simulink model "sampleModel2438"  (R2017a)
settings: Solver=VariableStepAuto  StartTime=0.0  StopTime=10.0  RelTol=1e-3
undefined symbols (not defined in the file or in its folder): DiscIntNeverNeededParam, sigbuilder_block
libraries: simulink x299
(part 1 of 5)
settings Model: Creator=cyfuzz  LastModifiedBy=cyfuzz

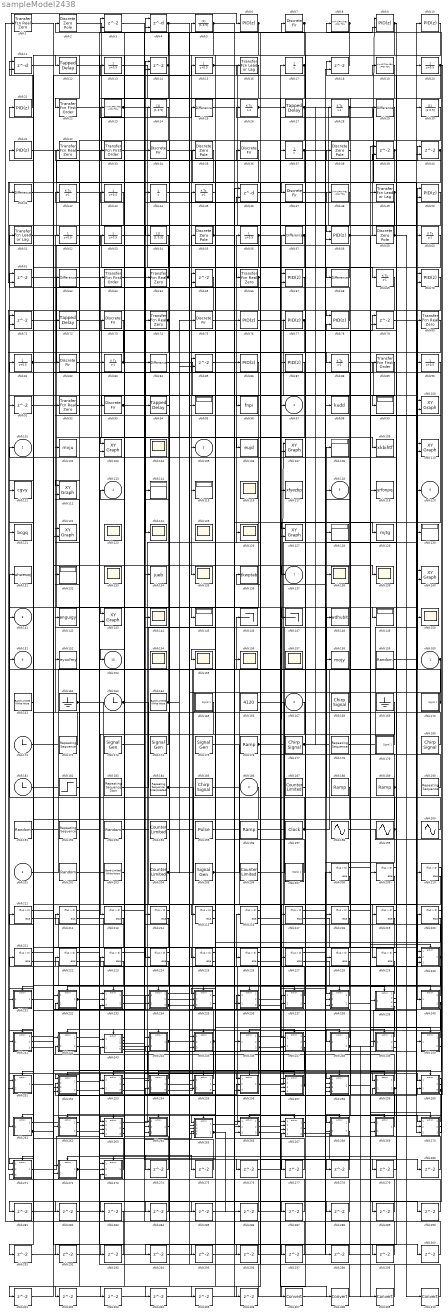
== system sampleModel2438 ==
  cfblk160 : Inport
  cfblk167 : Inport  Port=2
  cfblk186 : Inport  Port=3
  cfblk201 : Inport  Port=4
  cfblk{1,32,64,66,74,80,92} (7 alike) : simulink/Discrete/Transfer Fcn Real Zero  ZeroZ=0.75  ICPrevInput=0.0  DoSatur=off
      settings: SourceProductName=Simulink  SourceProductBaseCode=SL
  cfblk{6,10,21,31,76..77,86..87} (8 alike) : simulink/Continuous/PID Controller  Controller=PID  TimeDomain=Discrete-time  SampleTime=1  IntegratorMethod=Forward Euler  FilterMethod=Forward Euler  Form=Parallel  UseFilter=on  ControllerParametersSource=internal  P=1  I=1  D=0  N=100  InitialConditionSource=internal  InitialConditionForIntegrator=0  InitialConditionForFilter=0  ExternalReset=none  LimitOutput=off  UpperSaturationLimit=inf  LowerSaturationLimit=-inf  LinearizeAsGain=off  AntiWindupMode=none  Kb=1  TrackingMode=off  Kt=1  PParamMin=[]  PParamMax=[]  IParamMin=[]  IParamMax=[]  DParamMin=[]  DParamMax=[]  NParamMin=[]  NParamMax=[]  KbParamMin=[]  KbParamMax=[]  KtParamMin=[]  KtParamMax=[]  POutMin=[]  POutMax=[]  IOutMin=[]  IOutMax=[]  DOutMin=[]  DOutMax=[]  NOutMin=[]  NOutMax=[]  KbOutMin=[]  KbOutMax=[]  KtOutMin=[]  KtOutMax=[]  IntegratorOutMin=[]  IntegratorOutMax=[]  FilterOutMin=[]  FilterOutMax=[]  SumOutMin=[]  SumOutMax=[]  SumI1OutMin=[]  SumI1OutMax=[]  SumI2OutMin=[]  SumI2OutMax=[]  SumI3OutMin=[]  SumI3OutMax=[]  SumDOutMin=[]  SumDOutMax=[]  SaturationOutMin=[]  SaturationOutMax=[]  IntegratorContinuousStateAttributes=''  IntegratorStateMustResolveToSignalObject=off  IntegratorRTWStateStorageClass=Auto  FilterContinuousStateAttributes=''  FilterStateMustResolveToSignalObject=off  FilterRTWStateStorageClass=Auto  DifferentiatorICPrevScaledInput=0  DifferentiatorOutMin=[]  DifferentiatorOutMax=[]  InitialConditionSetting=State (most efficient)
  cfblk{100,103,107,110,112,122,127,140,143} (9 alike) : simulink/Sinks/XY Graph  xmin=-1  xmax=1  ymin=-1  ymax=1  st=-1
  cfblk102 : ToFile  Filename=mvju  SaveFormat=Timeseries
  cfblk{104,116,123..126,133,135,138..139,144,150,154..157} (16 alike) : Scope
      cfblk104 settings: Floating=on
      cfblk116 settings: Floating=on
      cfblk123 settings: Floating=on
      cfblk125 settings: Floating=on
      cfblk133 settings: Floating=on
      cfblk154 settings: Floating=on
      cfblk157 settings: Floating=on
  cfblk106 : ToFile  Filename=eujd  SaveFormat=Timeseries
  cfblk{95,99,108,114..115,128,130,132,145,149} (10 alike) : Display
  cfblk109 : ToWorkspace  VariableName=xkbihtf  SaveFormat=Timeseries  SampleTime=-1
  cfblk11 : Delay  DelayLengthSource=Input port  SampleTime=1
      settings: InputPortMap=u0,p1
  cfblk111 : ToFile  Filename=cgvy  SaveFormat=Timeseries
  cfblk117 : ToWorkspace  VariableName=xfyezbp  SaveFormat=Timeseries  SampleTime=-1
  cfblk119 : ToWorkspace  VariableName=yrfonpq  SaveFormat=Timeseries  SampleTime=-1
  cfblk{12,27,72,94} (4 alike) : simulink/Discrete/Tapped Delay  vinit=0.0  samptime=-1  NumDelays=1  DelayOrder=Oldest  includeCurrent=off
  cfblk121 : ToFile  Filename=bcgq  SaveFormat=Timeseries
  cfblk129 : ToFile  Filename=mjtg  SaveFormat=Timeseries
  cfblk{13,15,20,43,52..53,56,81,90} (9 alike) : DiscreteTransferFcn  SampleTime=1
  cfblk131 : ToWorkspace  VariableName=whweswj  SaveFormat=Timeseries  SampleTime=-1
  cfblk134 : ToFile  Filename=jueb  SaveFormat=Timeseries
  cfblk136 : ToWorkspace  VariableName=tkwpteb  SaveFormat=Timeseries  SampleTime=-1
  cfblk{3,14,18,39..40,61,65,71,79,85} (10 alike) : Delay  ShowEnablePort=on  SampleTime=1
      settings: InputPortMap=u0,e6
  cfblk142 : ToWorkspace  VariableName=enguigy  SaveFormat=Timeseries  SampleTime=-1
  cfblk146 : Terminator
  cfblk147 : Terminator
  cfblk148 : ToWorkspace  VariableName=wdhubit  SaveFormat=Timeseries  SampleTime=-1
  cfblk152 : ToWorkspace  VariableName=eyoxfmy  SaveFormat=Timeseries  SampleTime=-1
  cfblk158 : ToFile  Filename=mojy  SaveFormat=Timeseries
  cfblk{159,191,193,202} (4 alike) : UniformRandomNumber  SampleTime=0.1
  cfblk16 : simulink/Discrete/Transfer Fcn Lead or Lag  PoleZ=0.95  ZeroZ=0.75  ICPrevOutput=0.0  ICPrevInput=0.0  DoSatur=off
      settings: SourceProductName=Simulink  SourceProductBaseCode=SL
  cfblk161 : simulink/Sources/Band-Limited White Noise  Cov=[0.1]  Ts=0.1  seed=[23341]
  cfblk162 : Ground
  cfblk163 : Clock
  cfblk164 : simulink/Sources/Band-Limited White Noise  Cov=[0.1]  Ts=0.1  seed=[23341]
  cfblk165 : Subsystem  Tag=STV Subsys  LoadFcn=sigbuilder_block('load');  StartFcn=sigbuilder_block('start');  StopFcn=sigbuilder_block('stop');  ClipboardFcn=sigbuilder_block('clipboard');  mask(Sigbuilder block){tuvar=[0:10]}
      mask help: Simulink:masks:SigbuilderBlock_MD
      mask init:
      | if ~strcmp(get_param(bdroot(gcbh),'SimulationStatus'),'stopped') tuvar = sigbuilder_block('maskInit'); end
      settings: CopyFcn=sigbuilder_block('copy');  DeleteFcn=sigbuilder_block('delete');  ModelCloseFcn=sigbuilder_block('modelClose');  PreSaveFcn=sigbuilder_block('preSave');  PauseFcn=sigbuilder_block('pause');  ContinueFcn=sigbuilder_block('continue');  NameChangeFcn=sigbuilder_block('namechange');  OpenFcn=sigbuilder_block('open',[437.6 199.2 550.4 400 ]);  CloseFcn=sigbuilder_block('close');
      mask Display: plot(0, 0, 100, 100,[2, 2, 32, 32, 2], [68, 8, 8, 68, 68],[32, 2], [38, 38], [32, 19, 2],[53, 60, 44], [32, 17, 17, 2],[16, 16, 31, 31]);txt = getActiveGroup(gcbh);text(2, 100, txt,'verticalAlignment', 'top');
  cfblk166 : Constant  Value=4120
  cfblk{168,177,180,185} (4 alike) : simulink/Sources/Chirp Signal  f1=0.1  T=100  f2=1
  cfblk169 : Ground
  cfblk17 : UnitDelay
  cfblk170 : Subsystem  Tag=STV Subsys  LoadFcn=sigbuilder_block('load');  StartFcn=sigbuilder_block('start');  StopFcn=sigbuilder_block('stop');  ClipboardFcn=sigbuilder_block('clipboard');  mask(Sigbuilder block){tuvar=[0:10]}
      mask help: Simulink:masks:SigbuilderBlock_MD
      mask init:
      | if ~strcmp(get_param(bdroot(gcbh),'SimulationStatus'),'stopped') tuvar = sigbuilder_block('maskInit'); end
      settings: CopyFcn=sigbuilder_block('copy');  DeleteFcn=sigbuilder_block('delete');  ModelCloseFcn=sigbuilder_block('modelClose');  PreSaveFcn=sigbuilder_block('preSave');  PauseFcn=sigbuilder_block('pause');  ContinueFcn=sigbuilder_block('continue');  NameChangeFcn=sigbuilder_block('namechange');  OpenFcn=sigbuilder_block('open',[437.6 199.2 550.4 400 ]);  CloseFcn=sigbuilder_block('close');
      mask Display: plot(0, 0, 100, 100,[2, 2, 32, 32, 2], [68, 8, 8, 68, 68],[32, 2], [38, 38], [32, 19, 2],[53, 60, 44], [32, 17, 17, 2],[16, 16, 31, 31]);txt = getActiveGroup(gcbh);text(2, 100, txt,'verticalAlignment', 'top');
  cfblk171 : Clock
  cfblk{172,178,190,192} (4 alike) : simulink/Sources/Repeating Sequence  rep_seq_t=[0 2]  rep_seq_y=[0 2]
  cfblk{173..175,205} (4 alike) : SignalGenerator  Units=rad/sec
  cfblk{176,188..189,196} (4 alike) : simulink/Sources/Ramp  slope=1  start=0  X0=0
  cfblk179 : Subsystem  Tag=STV Subsys  LoadFcn=sigbuilder_block('load');  StartFcn=sigbuilder_block('start');  StopFcn=sigbuilder_block('stop');  ClipboardFcn=sigbuilder_block('clipboard');  mask(Sigbuilder block){tuvar=[0:10]}
      mask help: Simulink:masks:SigbuilderBlock_MD
      mask init:
      | if ~strcmp(get_param(bdroot(gcbh),'SimulationStatus'),'stopped') tuvar = sigbuilder_block('maskInit'); end
      settings: CopyFcn=sigbuilder_block('copy');  DeleteFcn=sigbuilder_block('delete');  ModelCloseFcn=sigbuilder_block('modelClose');  PreSaveFcn=sigbuilder_block('preSave');  PauseFcn=sigbuilder_block('pause');  ContinueFcn=sigbuilder_block('continue');  NameChangeFcn=sigbuilder_block('namechange');  OpenFcn=sigbuilder_block('open',[437.6 199.2 550.4 400 ]);  CloseFcn=sigbuilder_block('close');
      mask Display: plot(0, 0, 100, 100,[2, 2, 32, 32, 2], [68, 8, 8, 68, 68],[32, 2], [38, 38], [32, 19, 2],[53, 60, 44], [32, 17, 17, 2],[16, 16, 31, 31]);txt = getActiveGroup(gcbh);text(2, 100, txt,'verticalAlignment', 'top');
  cfblk181 : Clock
  cfblk182 : Step  After=81  SampleTime=0
  cfblk183 : simulink/Sources/Repeating Sequence Stair  OutValues=[3 1 4 2 1].'  tsamp=-1  OutMin=[]  OutMax=[]  OutDataTypeStr=double  OutputDataTypeScalingMode=double  OutDataType=fixdt(0,8)  ConRadixGroup=Best Precision: Vector-wise  OutScaling=2^-12
  cfblk184 : simulink/Sources/Repeating Sequence Interpolated  OutValues=[3 1 4 2 1].'  TimeValues=[0 0.1 0.5 0.6 1].'  LookUpMeth=Interpolation-Use End Values  tsamp=0.01  OutMin=[]  OutMax=[]  OutDataTypeStr=double  OutputDataTypeScalingMode=double  OutDataType=fixdt(0,8)  OutScaling=2^-10
  cfblk{187,194,204,206} (4 alike) : simulink/Sources/Counter Limited  uplimit=7  tsamp=-1
  cfblk{8,19,23,48} (4 alike) : DiscreteStateSpace
  cfblk195 : DiscretePulseGenerator  PulseType=Time based  Period=10  PulseWidth=5
  cfblk197 : DigitalClock
  cfblk198 : Sin  SampleTime=0
  cfblk199 : Sin  SampleTime=0
  cfblk{2,35,38,55,59} (5 alike) : DiscreteZeroPole  Poles=[0 0.5]  Gain=1
  cfblk200 : Sin  SampleTime=0
  cfblk203 : simulink/Sources/Band-Limited White Noise  Cov=[0.1]  Ts=0.1  seed=[23341]
  cfblk207 : Subsystem  Tag=STV Subsys  LoadFcn=sigbuilder_block('load');  StartFcn=sigbuilder_block('start');  StopFcn=sigbuilder_block('stop');  ClipboardFcn=sigbuilder_block('clipboard');  mask(Sigbuilder block){tuvar=[0:10]}
      mask help: Simulink:masks:SigbuilderBlock_MD
      mask init:
      | if ~strcmp(get_param(bdroot(gcbh),'SimulationStatus'),'stopped') tuvar = sigbuilder_block('maskInit'); end
      settings: CopyFcn=sigbuilder_block('copy');  DeleteFcn=sigbuilder_block('delete');  ModelCloseFcn=sigbuilder_block('modelClose');  PreSaveFcn=sigbuilder_block('preSave');  PauseFcn=sigbuilder_block('pause');  ContinueFcn=sigbuilder_block('continue');  NameChangeFcn=sigbuilder_block('namechange');  OpenFcn=sigbuilder_block('open',[437.6 199.2 550.4 400 ]);  CloseFcn=sigbuilder_block('close');
      mask Display: plot(0, 0, 100, 100,[2, 2, 32, 32, 2], [68, 8, 8, 68, 68],[32, 2], [38, 38], [32, 19, 2],[53, 60, 44], [32, 17, 17, 2],[16, 16, 31, 31]);txt = getActiveGroup(gcbh);text(2, 100, txt,'verticalAlignment', 'top');
  cfblk{208..229} (22 alike) : If  SampleTime=1
  cfblk{22,33,63,89} (4 alike) : simulink/Discrete/Transfer Fcn First Order  PoleZ=0.95  ICPrevOutput=0.0  DoSatur=off
      settings: SourceProductName=Simulink
  cfblk230 : Subsystem  TreatAsAtomicUnit=on
  cfblk231 : Subsystem  TreatAsAtomicUnit=on
  cfblk232 : Subsystem  TreatAsAtomicUnit=on
  cfblk233 : Subsystem  TreatAsAtomicUnit=on
  cfblk234 : Subsystem  TreatAsAtomicUnit=on
  cfblk235 : Subsystem  TreatAsAtomicUnit=on
  cfblk236 : Subsystem  TreatAsAtomicUnit=on
  cfblk237 : Subsystem  TreatAsAtomicUnit=on
  cfblk238 : Subsystem  TreatAsAtomicUnit=on
  cfblk239 : Subsystem  TreatAsAtomicUnit=on
  cfblk{5,24,30,54} (4 alike) : DiscreteFilter  SampleTime=1
  cfblk240 : Subsystem  TreatAsAtomicUnit=on
  cfblk241 : Subsystem  TreatAsAtomicUnit=on
  cfblk242 : Subsystem  TreatAsAtomicUnit=on
  cfblk243 : Subsystem  TreatAsAtomicUnit=on
  cfblk244 : Subsystem  TreatAsAtomicUnit=on
  cfblk245 : Subsystem  TreatAsAtomicUnit=on
  cfblk246 : Subsystem  TreatAsAtomicUnit=on
  cfblk247 : Subsystem  TreatAsAtomicUnit=on
  cfblk248 : Subsystem  TreatAsAtomicUnit=on
  cfblk249 : Subsystem  TreatAsAtomicUnit=on
  cfblk{25,29,41,57,62,68,84} (7 alike) : simulink/Discrete/Difference  ICPrevInput=0.0  OutMin=[]  OutMax=[]  OutDataTypeStr=Inherit: Inherit via back propagation  OutDataType=fixdt(1, 16)  OutScaling=2^-10  DoSatur=off
  cfblk250 : Subsystem  TreatAsAtomicUnit=on
  cfblk251 : Subsystem  TreatAsAtomicUnit=on
  cfblk252 : Subsystem  TreatAsAtomicUnit=on
  cfblk253 : Subsystem  TreatAsAtomicUnit=on
  cfblk254 : Subsystem  TreatAsAtomicUnit=on
  cfblk255 : Subsystem  TreatAsAtomicUnit=on
  cfblk256 : Subsystem  TreatAsAtomicUnit=on
  cfblk257 : Subsystem  TreatAsAtomicUnit=on
  cfblk258 : Subsystem  TreatAsAtomicUnit=on
  cfblk259 : Subsystem  TreatAsAtomicUnit=on
  cfblk{26,28,42,45,60,69,83,88} (8 alike) : DiscreteIntegrator  InitialConditionSetting=State (most efficient)  ICPrevOutput=DiscIntNeverNeededParam  ICPrevScaledInput=DiscIntNeverNeededParam
  cfblk260 : Subsystem  TreatAsAtomicUnit=on
  cfblk261 : Subsystem  TreatAsAtomicUnit=on
  cfblk262 : Subsystem  TreatAsAtomicUnit=on
  cfblk263 : Subsystem  TreatAsAtomicUnit=on
  cfblk264 : Subsystem  TreatAsAtomicUnit=on
  cfblk265 : Subsystem  TreatAsAtomicUnit=on
  cfblk266 : Subsystem  TreatAsAtomicUnit=on
  cfblk267 : Subsystem  TreatAsAtomicUnit=on
  cfblk268 : Subsystem  TreatAsAtomicUnit=on
  cfblk269 : Subsystem  TreatAsAtomicUnit=on
  cfblk270 : Subsystem  TreatAsAtomicUnit=on
  cfblk271 : Subsystem  TreatAsAtomicUnit=on
  cfblk272 : Subsystem  TreatAsAtomicUnit=on
  cfblk273 : Subsystem  TreatAsAtomicUnit=on
  cfblk{91,274..306} (34 alike) : Delay  SampleTime=1
  cfblk{307..310} (4 alike) : DataTypeConversion
  cfblk{7,34,36,47,73,75,82,93} (8 alike) : DiscreteFir  SampleTime=1
  cfblk37 : UnitDelay
  cfblk4 : Delay  DelayLengthSource=Input port  SampleTime=1
      settings: InputPortMap=u0,p1
  cfblk44 : UnitDelay
  cfblk46 : Delay  DelayLengthSource=Input port  SampleTime=1
      settings: InputPortMap=u0,p1
  cfblk49 : simulink/Discrete/Transfer Fcn Lead or Lag  PoleZ=0.95  ZeroZ=0.75  ICPrevOutput=0.0  ICPrevInput=0.0  DoSatur=off
      settings: SourceProductName=Simulink  SourceProductBaseCode=SL
  cfblk{9,50,58,67,70,78} (6 alike) : simulink/Continuous/PID Controller (2DOF)  Controller=PID  TimeDomain=Discrete-time  SampleTime=1  IntegratorMethod=Forward Euler  FilterMethod=Forward Euler  Form=Parallel  UseFilter=on  ControllerParametersSource=internal  P=1  I=1  D=0  N=100  b=1  c=1  InitialConditionSource=internal  InitialConditionForIntegrator=0  InitialConditionForFilter=0  ExternalReset=none  LimitOutput=off  UpperSaturationLimit=inf  LowerSaturationLimit=-inf  LinearizeAsGain=off  AntiWindupMode=none  Kb=1  TrackingMode=off  Kt=1  PParamMin=[]  PParamMax=[]  IParamMin=[]  IParamMax=[]  DParamMin=[]  DParamMax=[]  NParamMin=[]  NParamMax=[]  bParamMin=[]  bParamMax=[]  cParamMin=[]  cParamMax=[]  KbParamMin=[]  KbParamMax=[]  KtParamMin=[]  KtParamMax=[]  POutMin=[]  POutMax=[]  IOutMin=[]  IOutMax=[]  DOutMin=[]  DOutMax=[]  NOutMin=[]  NOutMax=[]  bOutMin=[]  bOutMax=[]  cOutMin=[]  cOutMax=[]  KbOutMin=[]  KbOutMax=[]  KtOutMin=[]  KtOutMax=[]  IntegratorOutMin=[]  IntegratorOutMax=[]  FilterOutMin=[]  FilterOutMax=[]  SumOutMin=[]  SumOutMax=[]  Sum1OutMin=[]  Sum1OutMax=[]  Sum2OutMin=[]  Sum2OutMax=[]  Sum3OutMin=[]  Sum3OutMax=[]  SumI1OutMin=[]  SumI1OutMax=[]  SumI2OutMin=[]  SumI2OutMax=[]  SumI3OutMin=[]  SumI3OutMax=[]  SumDOutMin=[]  SumDOutMax=[]  SaturationOutMin=[]  SaturationOutMax=[]  IntegratorContinuousStateAttributes=''  IntegratorStateMustResolveToSignalObject=off  IntegratorRTWStateStorageClass=Auto  FilterContinuousStateAttributes=''  FilterStateMustResolveToSignalObject=off  FilterRTWStateStorageClass=Auto  DifferentiatorICPrevScaledInput=0  DifferentiatorOutMin=[]  DifferentiatorOutMax=[]  InitialConditionSetting=State (most efficient)
  cfblk51 : simulink/Discrete/Transfer Fcn Lead or Lag  PoleZ=0.95  ZeroZ=0.75  ICPrevOutput=0.0  ICPrevInput=0.0  DoSatur=off
      settings: SourceProductName=Simulink  SourceProductBaseCode=SL
  cfblk96 : ToFile  Filename=fnpi  SaveFormat=Timeseries
  cfblk98 : ToFile  Filename=kudd  SaveFormat=Timeseries
  cfblk97 : Outport
  cfblk101 : Outport  Port=2
  cfblk105 : Outport  Port=3
  cfblk113 : Outport  Port=4
  cfblk118 : Outport  Port=5
  cfblk120 : Outport  Port=6
  cfblk137 : Outport  Port=7
  cfblk141 : Outport  Port=8
  cfblk151 : Outport  Port=9
  cfblk153 : Outport  Port=10
  wires:
  cfblk43/1 -> cfblk261/1(cfblk1)
  cfblk10/1 -> cfblk135/1
  cfblk246/1(cfblk2) -> cfblk259/1(cfblk1)
  cfblk200/1 -> cfblk108/1
  cfblk83/1 -> cfblk63/1, cfblk258/4(cfblk15)
  cfblk18/1 -> cfblk12/1
  cfblk238/1(cfblk2) -> cfblk14/1
  cfblk237/1(cfblk2) -> cfblk55/1
  cfblk198/1 -> cfblk50/1
  cfblk273/1(cfblk2) -> cfblk71/1
  cfblk58/1 -> cfblk9/1, cfblk230/3(cfblk14), cfblk290/1
  cfblk239/1(cfblk2) -> cfblk57/1
  cfblk45/1 -> cfblk145/1
  cfblk51/1 -> cfblk40/1
  cfblk16/1 -> cfblk155/1
  cfblk4/1 -> cfblk88/1, cfblk293/1
  cfblk194/1 -> cfblk50/2
  cfblk52/1 -> cfblk124/1
  cfblk23/1 -> cfblk69/1, cfblk258/1(cfblk1)
  cfblk239/2(cfblk14) -> cfblk71/2
  cfblk166/1 -> cfblk269/1(cfblk1)
  cfblk189/1 -> cfblk271/1(cfblk1), cfblk257/4(cfblk17), cfblk118/1
  cfblk195/1 -> cfblk97/1
  cfblk79/1 -> cfblk240/1(cfblk1)
  cfblk230/1(cfblk2) -> cfblk126/1, cfblk291/1
  cfblk176/1 -> cfblk107/1, cfblk230/2(cfblk13)
  cfblk261/1(cfblk2) -> cfblk210/1
  cfblk15/1 -> cfblk58/1, cfblk147/1
  cfblk180/1 -> cfblk52/1
  cfblk248/1(cfblk2) -> cfblk142/1
  cfblk14/1 -> cfblk2/1, cfblk264/3(cfblk7)
  cfblk50/1 -> cfblk241/1(cfblk1)
  cfblk174/1 -> cfblk3/1
  cfblk77/1 -> cfblk253/1(cfblk1), cfblk271/2(cfblk8)
  cfblk199/1 -> cfblk131/1, cfblk238/2(cfblk15)
  cfblk263/1(cfblk2) -> cfblk56/1
  cfblk87/1 -> cfblk103/1
  cfblk206/1 -> cfblk98/1
  cfblk168/1 -> cfblk81/1
  cfblk62/1 -> cfblk149/1
  cfblk57/1 -> cfblk143/1, cfblk66/1, cfblk106/1, cfblk292/1
  cfblk61/1 -> cfblk238/1(cfblk1)
  cfblk6/1 -> cfblk143/2, cfblk105/1
  cfblk244/1(cfblk2) -> cfblk40/2, cfblk227/1
  cfblk55/1 -> cfblk109/1, cfblk54/1
  cfblk84/1 -> cfblk100/1
  cfblk240/1(cfblk2) -> cfblk216/1
  cfblk80/1 -> cfblk225/1
  cfblk54/1 -> cfblk84/1
  cfblk91/1 -> cfblk103/2
  cfblk249/1(cfblk2) -> cfblk31/1
  cfblk24/1 -> cfblk112/1
  cfblk29/1 -> cfblk263/1(cfblk1)
  cfblk1/1 -> cfblk226/1
  cfblk90/1 -> cfblk127/1
  cfblk8/1 -> cfblk264/2(cfblk6), cfblk287/1
  cfblk197/1 -> cfblk20/1, cfblk36/1
  cfblk59/1 -> cfblk44/1, cfblk310/1
  cfblk258/1(cfblk2) -> cfblk260/1(cfblk1)
  cfblk163/1 -> cfblk250/1(cfblk1), cfblk217/1
  cfblk72/1 -> cfblk119/1
  cfblk181/1 -> cfblk148/1
  cfblk20/1 -> cfblk260/2(cfblk13), cfblk235/3(cfblk11)
  cfblk205/1 -> cfblk49/1, cfblk140/2
  cfblk265/1(cfblk2) -> cfblk70/1
  cfblk2/1 -> cfblk58/2
  cfblk167/1 -> cfblk213/1
  cfblk204/1 -> cfblk146/1, cfblk75/1, cfblk14/2
  cfblk172/1 -> cfblk51/1
  cfblk69/1 -> cfblk215/1
  cfblk86/1 -> cfblk141/1
  cfblk249/2(cfblk6) -> cfblk102/1
  cfblk171/1 -> cfblk76/1
  cfblk240/2(cfblk8) -> cfblk265/5(cfblk9), cfblk305/1
  cfblk32/1 -> cfblk24/1
  cfblk74/1 -> cfblk23/1, cfblk263/4(cfblk7)
  cfblk78/1 -> cfblk42/1
  cfblk269/1(cfblk2) -> cfblk73/1
  cfblk73/1 -> cfblk252/1(cfblk1)
  cfblk28/1 -> cfblk80/1, cfblk258/3(cfblk14)
  cfblk66/1 -> cfblk94/1, cfblk16/1
  cfblk177/1 -> cfblk10/1, cfblk28/1
  cfblk40/1 -> cfblk224/1, cfblk306/1
  cfblk250/1(cfblk2) -> cfblk128/1
  cfblk246/3(cfblk10) -> cfblk138/1, cfblk302/1
  cfblk60/1 -> cfblk121/1
  cfblk30/1 -> cfblk74/1
  cfblk255/1(cfblk2) -> cfblk101/1
  cfblk11/1 -> cfblk139/1
  cfblk38/1 -> cfblk78/1
  cfblk261/2(cfblk11) -> cfblk270/1(cfblk1), cfblk89/1
  cfblk94/1 -> cfblk64/1
  cfblk183/1 -> cfblk39/1
  cfblk256/1(cfblk2) -> cfblk110/1, cfblk72/1
  cfblk185/1 -> cfblk247/1(cfblk1)
  cfblk68/1 -> cfblk45/1
  cfblk182/1 -> cfblk112/2
  cfblk21/1 -> cfblk6/1
  cfblk268/1(cfblk2) -> cfblk252/2(cfblk12)
  cfblk92/1 -> cfblk96/1
  cfblk196/1 -> cfblk218/1
  cfblk89/1 -> cfblk91/1
  cfblk254/1(cfblk2) -> cfblk251/1(cfblk1)
  cfblk165/1(Signal 1) -> cfblk233/2(cfblk13)
  cfblk264/1(cfblk2) -> cfblk114/1
  cfblk257/1(cfblk2) -> cfblk212/1, cfblk151/1
  cfblk233/1(cfblk2) -> cfblk220/1
  cfblk81/1 -> cfblk17/1, cfblk15/1
  cfblk270/1(cfblk2) -> cfblk234/1(cfblk1)
  cfblk255/2(cfblk9) -> cfblk273/2(cfblk9)
  cfblk27/1 -> cfblk270/2(cfblk9), cfblk245/3(cfblk9)
  cfblk233/2(cfblk15) -> cfblk78/2
  cfblk249/3(cfblk7) -> cfblk38/1
  cfblk85/1 -> cfblk156/1
  cfblk253/1(cfblk2) -> cfblk90/1
  cfblk75/1 -> cfblk129/1
  cfblk37/1 -> cfblk150/1, cfblk272/2(cfblk10)
  cfblk250/2(cfblk10) -> cfblk34/1
  cfblk248/2(cfblk11) -> cfblk30/1, cfblk309/1
  cfblk12/1 -> cfblk95/1
  cfblk93/1 -> cfblk107/2, cfblk258/2(cfblk13)
  cfblk186/1 -> cfblk235/1(cfblk1)
  cfblk259/1(cfblk2) -> cfblk242/2(cfblk9)
  cfblk190/1 -> cfblk136/1
  cfblk201/1 -> cfblk120/1
  cfblk71/1 -> cfblk115/1
  cfblk64/1 -> cfblk4/1, cfblk11/1
  cfblk259/2(cfblk8) -> cfblk236/1(cfblk1), cfblk268/2(cfblk7)
  cfblk5/1 -> cfblk252/3(cfblk13), cfblk300/1
  cfblk173/1 -> cfblk134/1
  cfblk245/1(cfblk2) -> cfblk122/1, cfblk263/3(cfblk6)
  cfblk184/1 -> cfblk130/1, cfblk18/2, cfblk219/1
  cfblk232/1(cfblk2) -> cfblk79/1, cfblk4/2
  cfblk192/1 -> cfblk83/1
  cfblk179/1(Signal 1) -> cfblk132/1
  cfblk35/1 -> cfblk41/1
  cfblk48/1 -> cfblk122/2
  cfblk161/1 -> cfblk21/1
  cfblk254/2(cfblk12) -> cfblk256/1(cfblk1)
  cfblk160/1 -> cfblk236/2(cfblk10), cfblk265/3(cfblk7)
  cfblk191/1 -> cfblk27/1
  cfblk76/1 -> cfblk99/1
  cfblk254/3(cfblk13) -> cfblk37/1
  cfblk26/1 -> cfblk248/1(cfblk1), cfblk270/3(cfblk10)
  cfblk7/1 -> cfblk22/1, cfblk256/3(cfblk17)
  cfblk202/1 -> cfblk257/1(cfblk1)
  cfblk33/1 -> cfblk47/1
  cfblk262/1(cfblk2) -> cfblk232/2(cfblk8)
  cfblk267/2(cfblk13) -> cfblk3/2
  cfblk271/1(cfblk2) -> cfblk256/2(cfblk16)
  cfblk237/2(cfblk10) -> cfblk62/1
  cfblk236/1(cfblk2) -> cfblk221/1
  cfblk39/1 -> cfblk127/2, cfblk61/2
  cfblk49/1 -> cfblk228/1, cfblk252/4(cfblk14)
  cfblk169/1 -> cfblk257/2(cfblk15)
  cfblk252/1(cfblk2) -> cfblk67/1
  cfblk88/1 -> cfblk110/2
  cfblk13/1 -> cfblk86/1
  cfblk9/1 -> cfblk231/1(cfblk1), cfblk289/1
  cfblk193/1 -> cfblk255/1(cfblk1)
  cfblk239/4(cfblk16) -> cfblk268/1(cfblk1)
  cfblk265/2(cfblk10) -> cfblk285/1, cfblk286/1
  cfblk236/2(cfblk11) -> cfblk237/1(cfblk1)
  cfblk162/1 -> cfblk229/1, cfblk245/1(cfblk1)
  cfblk36/1 -> cfblk235/2(cfblk10)
  cfblk63/1 -> cfblk9/2
  cfblk188/1 -> cfblk255/2(cfblk8)
  cfblk53/1 -> cfblk117/1
  cfblk272/1(cfblk2) -> cfblk25/1, cfblk265/4(cfblk8)
  cfblk175/1 -> cfblk269/2(cfblk10)
  cfblk203/1 -> cfblk113/1
  cfblk17/1 -> cfblk253/2(cfblk15), cfblk267/3(cfblk11)
  cfblk266/1(cfblk2) -> cfblk26/1
  cfblk263/2(cfblk8) -> cfblk152/1
  cfblk251/1(cfblk2) -> cfblk234/2(cfblk13)
  cfblk34/1 -> cfblk60/1
  cfblk247/1(cfblk2) -> cfblk77/1
  cfblk263/3(cfblk9) -> cfblk53/1
  cfblk253/3(cfblk17) -> cfblk85/1
  cfblk67/1 -> cfblk251/2(cfblk9)
  cfblk31/1 -> cfblk264/1(cfblk1)
  cfblk238/2(cfblk17) -> cfblk100/2
  cfblk19/1 -> cfblk68/1
  cfblk247/2(cfblk16) -> cfblk13/1
  cfblk65/1 -> cfblk111/1
  cfblk164/1 -> cfblk32/1, cfblk85/2
  cfblk235/2(cfblk12) -> cfblk144/1
  cfblk44/1 -> cfblk137/1
  cfblk260/2(cfblk14) -> cfblk265/1(cfblk1)
  cfblk207/1(Signal 1) -> cfblk65/1
  cfblk242/2(cfblk10) -> cfblk230/1(cfblk1)
  cfblk56/1 -> cfblk153/1, cfblk238/3(cfblk16)
  cfblk159/1 -> cfblk70/2
  cfblk231/1(cfblk2) -> cfblk87/1
  cfblk262/2(cfblk7) -> cfblk93/1
  cfblk243/2(cfblk14) -> cfblk43/1
  cfblk234/1(cfblk2) -> cfblk7/1
  cfblk255/3(cfblk10) -> cfblk33/1
  cfblk266/2(cfblk15) -> cfblk247/2(cfblk15)
  cfblk241/1(cfblk2) -> cfblk265/2(cfblk6)
  cfblk266/3(cfblk16) -> cfblk29/1, cfblk61/1
  cfblk270/2(cfblk11) -> cfblk82/1
  cfblk260/3(cfblk15) -> cfblk8/1, cfblk18/1
  cfblk270/3(cfblk12) -> cfblk92/1
  cfblk178/1 -> cfblk140/1
  cfblk243/3(cfblk15) -> cfblk65/2
  cfblk241/2(cfblk7) -> cfblk67/2
  cfblk243/4(cfblk16) -> cfblk257/3(cfblk16)
  cfblk243/5(cfblk17) -> cfblk35/1
  cfblk241/3(cfblk8) -> cfblk272/1(cfblk1)
  cfblk170/1(Signal 1) -> cfblk158/1, cfblk11/2, cfblk19/1
  cfblk234/2(cfblk14) -> cfblk237/2(cfblk9)
  cfblk234/3(cfblk15) -> cfblk48/1, cfblk276/1
  cfblk236/3(cfblk12) -> cfblk39/2, cfblk5/1
  cfblk208/1 -> cfblk230/Action
  cfblk208/2 -> cfblk231/Action
  cfblk209/1 -> cfblk232/Action
  cfblk209/2 -> cfblk233/Action
  cfblk210/1 -> cfblk234/Action
  cfblk210/2 -> cfblk235/Action
  cfblk211/1 -> cfblk236/Action
  cfblk211/2 -> cfblk237/Action
  cfblk212/1 -> cfblk238/Action
  cfblk212/2 -> cfblk239/Action
  cfblk213/1 -> cfblk240/Action
  cfblk213/2 -> cfblk241/Action
  cfblk214/1 -> cfblk242/Action
  cfblk214/2 -> cfblk243/Action
  cfblk215/1 -> cfblk244/Action
  cfblk215/2 -> cfblk245/Action
  cfblk216/1 -> cfblk246/Action
  cfblk216/2 -> cfblk247/Action
  cfblk217/1 -> cfblk248/Action
  cfblk217/2 -> cfblk249/Action
  cfblk218/1 -> cfblk250/Action
  cfblk218/2 -> cfblk251/Action
  cfblk219/1 -> cfblk252/Action
  cfblk219/2 -> cfblk253/Action
  cfblk220/1 -> cfblk254/Action
  cfblk220/2 -> cfblk255/Action
  cfblk221/1 -> cfblk256/Action
  cfblk221/2 -> cfblk257/Action
  cfblk222/1 -> cfblk258/Action
  cfblk222/2 -> cfblk259/Action
  cfblk223/1 -> cfblk260/Action
  cfblk223/2 -> cfblk261/Action
  cfblk224/1 -> cfblk262/Action
  cfblk224/2 -> cfblk263/Action
  cfblk225/1 -> cfblk264/Action
  cfblk225/2 -> cfblk265/Action
  cfblk226/1 -> cfblk266/Action
  cfblk226/2 -> cfblk267/Action
  cfblk227/1 -> cfblk268/Action
  cfblk227/2 -> cfblk269/Action
  cfblk228/1 -> cfblk270/Action
  cfblk228/2 -> cfblk271/Action
  cfblk229/1 -> cfblk272/Action
  cfblk229/2 -> cfblk273/Action
  cfblk242/1(cfblk2) -> cfblk274/1
  cfblk274/1 -> cfblk233/3(cfblk14)
  cfblk22/1 -> cfblk275/1
  cfblk275/1 -> cfblk244/1(cfblk1)
  cfblk276/1 -> cfblk267/4(cfblk12)
  cfblk267/1(cfblk2) -> cfblk277/1
  cfblk277/1 -> cfblk232/1(cfblk1)
  cfblk3/1 -> cfblk278/1
  cfblk278/1 -> cfblk242/1(cfblk1)
  cfblk267/3(cfblk14) -> cfblk279/1
  cfblk279/1 -> cfblk259/2(cfblk7)
  cfblk25/1 -> cfblk280/1
  cfblk280/1 -> cfblk243/2(cfblk13)
  cfblk243/1(cfblk2) -> cfblk281/1
  cfblk281/1 -> cfblk266/3(cfblk14)
  cfblk235/1(cfblk2) -> cfblk282/1
  cfblk282/1 -> cfblk267/2(cfblk10)
  cfblk260/1(cfblk2) -> cfblk283/1
  cfblk283/1 -> cfblk1/1
  cfblk70/1 -> cfblk284/1
  cfblk284/1 -> cfblk273/1(cfblk1)
  cfblk285/1 -> cfblk266/2(cfblk13)
  cfblk286/1 -> cfblk271/3(cfblk9)
  cfblk287/1 -> cfblk214/1
  cfblk82/1 -> cfblk288/1
  cfblk288/1 -> cfblk223/1
  cfblk289/1 -> cfblk273/3(cfblk10)
  cfblk290/1 -> cfblk244/2(cfblk7)
  cfblk291/1 -> cfblk239/1(cfblk1)
  cfblk292/1 -> cfblk246/1(cfblk1)
  cfblk293/1 -> cfblk243/1(cfblk1)
  cfblk239/3(cfblk15) -> cfblk294/1
  cfblk294/1 -> cfblk209/1
  cfblk252/2(cfblk15) -> cfblk295/1
  cfblk295/1 -> cfblk208/1
  cfblk268/2(cfblk8) -> cfblk296/1
  cfblk296/1 -> cfblk254/1(cfblk1)
  cfblk41/1 -> cfblk297/1
  cfblk297/1 -> cfblk254/2(cfblk11)
  cfblk47/1 -> cfblk298/1
  cfblk298/1 -> cfblk233/1(cfblk1)
  cfblk42/1 -> cfblk299/1
  cfblk299/1 -> cfblk222/1
  cfblk300/1 -> cfblk211/1
  cfblk246/2(cfblk9) -> cfblk301/1
  cfblk301/1 -> cfblk262/1(cfblk1)
  cfblk302/1 -> cfblk249/1(cfblk1)
  cfblk253/2(cfblk16) -> cfblk303/1
  cfblk303/1 -> cfblk267/1(cfblk1)
  cfblk247/3(cfblk17) -> cfblk304/1
  cfblk304/1 -> cfblk79/2
  cfblk305/1 -> cfblk266/1(cfblk1)
  cfblk306/1 -> cfblk245/2(cfblk8)
  cfblk187/1 -> cfblk307/1
  cfblk307/1 -> cfblk59/1
  cfblk46/1 -> cfblk308/1
  cfblk308/1 -> cfblk263/2(cfblk5)
  cfblk309/1 -> cfblk46/1
  cfblk310/1 -> cfblk46/2

== system sampleModel2438/cfblk165 ==
  Demux : Demux  Tag=STV Demux  Outputs=1
  FromWs : FromWorkspace  Tag=STV FromWs  VariableName=tuvar  SampleTime=0
      SigBuilderData=|
      | common.afterFinalStr = 'Extrapolate'
      | common.sampleTime = 0
      | dataSet.timeRange = [0 10]
      | dataSet.name = 'Group 1'
      | sbobj.Groups.Name = 'Group 1'
      | sbobj.Groups.Signals.Name = 'Signal 1'
      | sbobj.Groups.Signals.XData = [0 4 4 6 6 10]
      | sbobj.Groups.Signals.YData = [0 0 1 1 0 0]
  Signal 1 : Outport  Tag=STV Outport
  wires:
  Demux/1 -> Signal 1/1
  FromWs/1 -> Demux/1

== system sampleModel2438/cfblk170 ==
  Demux : Demux  Tag=STV Demux  Outputs=1
  FromWs : FromWorkspace  Tag=STV FromWs  VariableName=tuvar  SampleTime=0
      SigBuilderData=|
      | common.afterFinalStr = 'Extrapolate'
      | common.sampleTime = 0
      | dataSet.timeRange = [0 10]
      | dataSet.name = 'Group 1'
      | sbobj.Groups.Name = 'Group 1'
      | sbobj.Groups.Signals.Name = 'Signal 1'
      | sbobj.Groups.Signals.XData = [0 4 4 6 6 10]
      | sbobj.Groups.Signals.YData = [0 0 1 1 0 0]
  Signal 1 : Outport  Tag=STV Outport
  wires:
  Demux/1 -> Signal 1/1
  FromWs/1 -> Demux/1

== system sampleModel2438/cfblk179 ==
  Demux : Demux  Tag=STV Demux  Outputs=1
  FromWs : FromWorkspace  Tag=STV FromWs  VariableName=tuvar  SampleTime=0
      SigBuilderData=|
      | common.afterFinalStr = 'Extrapolate'
      | common.sampleTime = 0
      | dataSet.timeRange = [0 10]
      | dataSet.name = 'Group 1'
      | sbobj.Groups.Name = 'Group 1'
      | sbobj.Groups.Signals.Name = 'Signal 1'
      | sbobj.Groups.Signals.XData = [0 4 4 6 6 10]
      | sbobj.Groups.Signals.YData = [0 0 1 1 0 0]
  Signal 1 : Outport  Tag=STV Outport
  wires:
  Demux/1 -> Signal 1/1
  FromWs/1 -> Demux/1

== system sampleModel2438/cfblk207 ==
  Demux : Demux  Tag=STV Demux  Outputs=1
  FromWs : FromWorkspace  Tag=STV FromWs  VariableName=tuvar  SampleTime=0
      SigBuilderData=|
      | common.afterFinalStr = 'Extrapolate'
      | common.sampleTime = 0
      | dataSet.timeRange = [0 10]
      | dataSet.name = 'Group 1'
      | sbobj.Groups.Name = 'Group 1'
      | sbobj.Groups.Signals.Name = 'Signal 1'
      | sbobj.Groups.Signals.XData = [0 4 4 6 6 10]
      | sbobj.Groups.Signals.YData = [0 0 1 1 0 0]
  Signal 1 : Outport  Tag=STV Outport
  wires:
  Demux/1 -> Signal 1/1
  FromWs/1 -> Demux/1

== system sampleModel2438/cfblk230 ==
  cfblk1 : Inport
  cfblk13 : Inport  Port=2
  cfblk14 : Inport  Port=3
  Action Port : ActionPort  ActionType=then
  cfblk10 : UnitDelay  SampleTime=-1
  cfblk11 : DiscreteIntegrator  InitialConditionSetting=State (most efficient)  SampleTime=-1  ICPrevOutput=DiscIntNeverNeededParam  ICPrevScaledInput=DiscIntNeverNeededParam
  cfblk12 : simulink/Discrete/Transfer Fcn Lead or Lag  PoleZ=0.95  ZeroZ=0.75  ICPrevOutput=0.0  ICPrevInput=0.0  DoSatur=off
      settings: SourceProductName=Simulink  SourceProductBaseCode=SL
  cfblk15 : Delay
  cfblk3 : Delay  ShowEnablePort=on
      settings: InputPortMap=u0,e6
  cfblk4 : Delay
  cfblk5 : DiscreteFilter
  cfblk6 : Delay  DelayLengthSource=Input port
      settings: InputPortMap=u0,p1
  cfblk7 : DiscreteZeroPole  Poles=[0 0.5]  Gain=1  SampleTime=-1
  cfblk8 : DiscreteZeroPole  Poles=[0 0.5]  Gain=1  SampleTime=-1
  cfblk9 : UnitDelay  SampleTime=-1
  cfblk2 : Outport
  wires:
  cfblk1/1 -> cfblk4/1
  cfblk11/1 -> cfblk7/1
  cfblk8/1 -> cfblk10/1
  cfblk5/1 -> cfblk6/1
  cfblk3/1 -> cfblk9/1
  cfblk12/1 -> cfblk5/1
  cfblk14/1 -> cfblk8/1
  cfblk13/1 -> cfblk6/2
  cfblk10/1 -> cfblk11/1
  cfblk4/1 -> cfblk12/1
  cfblk6/1 -> cfblk3/1
  cfblk7/1 -> cfblk2/1
  cfblk9/1 -> cfblk15/1
  cfblk15/1 -> cfblk3/2

== system sampleModel2438/cfblk231 ==
  cfblk1 : Inport
  Action Port : ActionPort  ActionType=else
  cfblk10 : Delay
  cfblk3 : simulink/Discrete/Difference  ICPrevInput=0.0  OutMin=[]  OutMax=[]  OutDataTypeStr=Inherit: Inherit via back propagation  OutDataType=fixdt(1, 16)  OutScaling=2^-10  DoSatur=off
  cfblk4 : DiscreteIntegrator  InitialConditionSetting=State (most efficient)  SampleTime=-1  ICPrevOutput=DiscIntNeverNeededParam  ICPrevScaledInput=DiscIntNeverNeededParam
  cfblk5 : Delay  ShowEnablePort=on
      settings: InputPortMap=u0,e6
  cfblk6 : Delay  ShowEnablePort=on
      settings: InputPortMap=u0,e6
  cfblk7 : DiscreteTransferFcn
  cfblk8 : Delay
  cfblk9 : DiscreteStateSpace  SampleTime=-1
  cfblk2 : Outport
  wires:
  cfblk6/1 -> cfblk2/1
  cfblk1/1 -> cfblk6/1, cfblk4/1, cfblk7/1
  cfblk4/1 -> cfblk3/1
  cfblk3/1 -> cfblk6/2
  cfblk5/1 -> cfblk8/1
  cfblk7/1 -> cfblk9/1
  cfblk9/1 -> cfblk5/2
  cfblk8/1 -> cfblk10/1
  cfblk10/1 -> cfblk5/1

== system sampleModel2438/cfblk232 ==
  cfblk1 : Inport
  cfblk8 : Inport  Port=2
  Action Port : ActionPort  ActionType=then
  cfblk10 : Subsystem  TreatAsAtomicUnit=on
  cfblk11 : Delay
  cfblk12 : Delay
  cfblk3 : Delay
  cfblk4 : simulink/Discrete/Transfer Fcn Lead or Lag  PoleZ=0.95  ZeroZ=0.75  ICPrevOutput=0.0  ICPrevInput=0.0  DoSatur=off
      settings: SourceProductName=Simulink  SourceProductBaseCode=SL
  cfblk5 : simulink/Discrete/Tapped Delay  vinit=0.0  samptime=-1  NumDelays=1  DelayOrder=Oldest  includeCurrent=off
  cfblk6 : simulink/Discrete/Tapped Delay  vinit=0.0  samptime=-1  NumDelays=1  DelayOrder=Oldest  includeCurrent=off
  cfblk7 : If  SampleTime=1
  cfblk9 : Subsystem  TreatAsAtomicUnit=on
  cfblk2 : Outport
  wires:
  cfblk4/1 -> cfblk2/1
  cfblk8/1 -> cfblk7/1
  cfblk1/1 -> cfblk9/2(cfblk9)
  cfblk10/2(cfblk10) -> cfblk6/1
  cfblk3/1 -> cfblk4/1
  cfblk6/1 -> cfblk5/1
  cfblk9/1(cfblk2) -> cfblk3/1
  cfblk9/2(cfblk11) -> cfblk10/1(cfblk1)
  cfblk9/3(cfblk12) -> cfblk10/2(cfblk8), cfblk10/3(cfblk9)
  cfblk7/1 -> cfblk9/Action
  cfblk7/2 -> cfblk10/Action
  cfblk10/1(cfblk2) -> cfblk11/1
  cfblk11/1 -> cfblk9/3(cfblk10)
  cfblk5/1 -> cfblk12/1
  cfblk12/1 -> cfblk9/1(cfblk1)

== system sampleModel2438/cfblk233 ==
  cfblk1 : Inport
  cfblk13 : Inport  Port=2
  cfblk14 : Inport  Port=3
  Action Port : ActionPort  ActionType=else
  cfblk10 : DiscreteStateSpace  SampleTime=-1
  cfblk11 : simulink/Discrete/Tapped Delay  vinit=0.0  samptime=-1  NumDelays=1  DelayOrder=Oldest  includeCurrent=off
  cfblk12 : simulink/Discrete/Transfer Fcn First Order  PoleZ=0.95  ICPrevOutput=0.0  DoSatur=off
      settings: SourceProductName=Simulink
  cfblk16 : Delay
  cfblk17 : Delay
  cfblk3 : DiscreteZeroPole  Poles=[0 0.5]  Gain=1  SampleTime=-1
  cfblk4 : Delay  DelayLengthSource=Input port
      settings: InputPortMap=u0,p1
  cfblk5 : Delay
  cfblk6 : Delay  ShowEnablePort=on
      settings: InputPortMap=u0,e6
  cfblk7 : DiscreteIntegrator  InitialConditionSetting=State (most efficient)  SampleTime=-1  ICPrevOutput=DiscIntNeverNeededParam  ICPrevScaledInput=DiscIntNeverNeededParam
  cfblk8 : simulink/Discrete/Transfer Fcn First Order  PoleZ=0.95  ICPrevOutput=0.0  DoSatur=off
      settings: SourceProductName=Simulink
  cfblk9 : DiscreteTransferFcn
  cfblk2 : Outport
  cfblk15 : Outport  Port=2
  wires:
  cfblk3/1 -> cfblk6/1
  cfblk6/1 -> cfblk8/1
  cfblk12/1 -> cfblk4/2
  cfblk10/1 -> cfblk3/1
  cfblk13/1 -> cfblk5/1
  cfblk11/1 -> cfblk15/1
  cfblk5/1 -> cfblk10/1
  cfblk9/1 -> cfblk11/1
  cfblk14/1 -> cfblk12/1
  cfblk4/1 -> cfblk7/1
  cfblk8/1 -> cfblk9/1, cfblk16/1
  cfblk1/1 -> cfblk2/1
  cfblk16/1 -> cfblk6/2
  cfblk7/1 -> cfblk17/1
  cfblk17/1 -> cfblk4/1

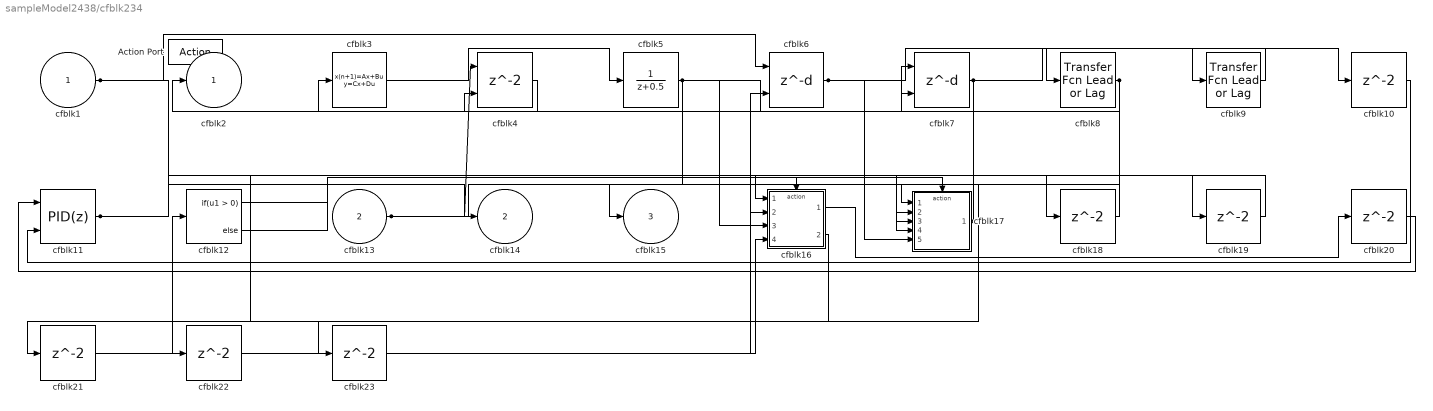
== system sampleModel2438/cfblk234 ==
  cfblk1 : Inport
  cfblk13 : Inport  Port=2
  Action Port : ActionPort  ActionType=then
  cfblk{10,18..23} (7 alike) : Delay
  cfblk11 : simulink/Continuous/PID Controller (2DOF)  Controller=PID  TimeDomain=Discrete-time  SampleTime=-1  IntegratorMethod=Forward Euler  FilterMethod=Forward Euler  Form=Parallel  UseFilter=on  ControllerParametersSource=internal  P=1  I=1  D=0  N=100  b=1  c=1  InitialConditionSource=internal  InitialConditionForIntegrator=0  InitialConditionForFilter=0  ExternalReset=none  LimitOutput=off  UpperSaturationLimit=inf  LowerSaturationLimit=-inf  LinearizeAsGain=off  AntiWindupMode=none  Kb=1  TrackingMode=off  Kt=1  PParamMin=[]  PParamMax=[]  IParamMin=[]  IParamMax=[]  DParamMin=[]  DParamMax=[]  NParamMin=[]  NParamMax=[]  bParamMin=[]  bParamMax=[]  cParamMin=[]  cParamMax=[]  KbParamMin=[]  KbParamMax=[]  KtParamMin=[]  KtParamMax=[]  POutMin=[]  POutMax=[]  IOutMin=[]  IOutMax=[]  DOutMin=[]  DOutMax=[]  NOutMin=[]  NOutMax=[]  bOutMin=[]  bOutMax=[]  cOutMin=[]  cOutMax=[]  KbOutMin=[]  KbOutMax=[]  KtOutMin=[]  KtOutMax=[]  IntegratorOutMin=[]  IntegratorOutMax=[]  FilterOutMin=[]  FilterOutMax=[]  SumOutMin=[]  SumOutMax=[]  Sum1OutMin=[]  Sum1OutMax=[]  Sum2OutMin=[]  Sum2OutMax=[]  Sum3OutMin=[]  Sum3OutMax=[]  SumI1OutMin=[]  SumI1OutMax=[]  SumI2OutMin=[]  SumI2OutMax=[]  SumI3OutMin=[]  SumI3OutMax=[]  SumDOutMin=[]  SumDOutMax=[]  SaturationOutMin=[]  SaturationOutMax=[]  IntegratorContinuousStateAttributes=''  IntegratorStateMustResolveToSignalObject=off  IntegratorRTWStateStorageClass=Auto  FilterContinuousStateAttributes=''  FilterStateMustResolveToSignalObject=off  FilterRTWStateStorageClass=Auto  DifferentiatorICPrevScaledInput=0  DifferentiatorOutMin=[]  DifferentiatorOutMax=[]  InitialConditionSetting=State (most efficient)
  cfblk12 : If  SampleTime=1
  cfblk16 : Subsystem  TreatAsAtomicUnit=on
  cfblk17 : Subsystem  TreatAsAtomicUnit=on
  cfblk3 : DiscreteStateSpace  SampleTime=-1
  cfblk4 : Delay  ShowEnablePort=on
      settings: InputPortMap=u0,e6
  cfblk5 : DiscreteTransferFcn
  cfblk6 : Delay  DelayLengthSource=Input port
      settings: InputPortMap=u0,p1
  cfblk7 : Delay  DelayLengthSource=Input port
      settings: InputPortMap=u0,p1
  cfblk8 : simulink/Discrete/Transfer Fcn Lead or Lag  PoleZ=0.95  ZeroZ=0.75  ICPrevOutput=0.0  ICPrevInput=0.0  DoSatur=off
      settings: SourceProductName=Simulink  SourceProductBaseCode=SL
  cfblk9 : simulink/Discrete/Transfer Fcn Lead or Lag  PoleZ=0.95  ZeroZ=0.75  ICPrevOutput=0.0  ICPrevInput=0.0  DoSatur=off
      settings: SourceProductName=Simulink  SourceProductBaseCode=SL
  cfblk2 : Outport
  cfblk14 : Outport  Port=2
  cfblk15 : Outport  Port=3
  wires:
  cfblk6/1 -> cfblk9/1, cfblk17/5(cfblk12)
  cfblk3/1 -> cfblk5/1
  cfblk17/1(cfblk2) -> cfblk7/1, cfblk2/1
  cfblk8/1 -> cfblk17/1(cfblk1), cfblk16/2(cfblk11), cfblk4/2, cfblk17/4(cfblk11), cfblk23/1
  cfblk4/1 -> cfblk3/1
  cfblk9/1 -> cfblk8/1
  cfblk7/1 -> cfblk10/1, cfblk22/1
  cfblk10/1 -> cfblk11/2
  cfblk13/1 -> cfblk4/1, cfblk17/3(cfblk10)
  cfblk1/1 -> cfblk6/1, cfblk14/1
  cfblk5/1 -> cfblk7/2, cfblk16/3(cfblk12), cfblk15/1
  cfblk11/1 -> cfblk18/1, cfblk19/1
  cfblk12/1 -> cfblk16/Action
  cfblk12/2 -> cfblk17/Action
  cfblk18/1 -> cfblk17/2(cfblk9)
  cfblk19/1 -> cfblk16/1(cfblk1)
  cfblk16/1(cfblk2) -> cfblk20/1
  cfblk20/1 -> cfblk11/1
  cfblk16/2(cfblk14) -> cfblk21/1
  cfblk21/1 -> cfblk12/1
  cfblk22/1 -> cfblk16/4(cfblk13)
  cfblk23/1 -> cfblk6/2

== system sampleModel2438/cfblk235 ==
  cfblk1 : Inport
  cfblk10 : Inport  Port=2
  cfblk11 : Inport  Port=3
  Action Port : ActionPort  ActionType=else
  cfblk13 : Subsystem  TreatAsAtomicUnit=on
  cfblk14 : Subsystem  TreatAsAtomicUnit=on
  cfblk{3,15..17} (4 alike) : Delay
  cfblk4 : simulink/Discrete/Tapped Delay  vinit=0.0  samptime=-1  NumDelays=1  DelayOrder=Oldest  includeCurrent=off
  cfblk5 : simulink/Continuous/PID Controller  Controller=PID  TimeDomain=Discrete-time  SampleTime=-1  IntegratorMethod=Forward Euler  FilterMethod=Forward Euler  Form=Parallel  UseFilter=on  ControllerParametersSource=internal  P=1  I=1  D=0  N=100  InitialConditionSource=internal  InitialConditionForIntegrator=0  InitialConditionForFilter=0  ExternalReset=none  LimitOutput=off  UpperSaturationLimit=inf  LowerSaturationLimit=-inf  LinearizeAsGain=off  AntiWindupMode=none  Kb=1  TrackingMode=off  Kt=1  PParamMin=[]  PParamMax=[]  IParamMin=[]  IParamMax=[]  DParamMin=[]  DParamMax=[]  NParamMin=[]  NParamMax=[]  KbParamMin=[]  KbParamMax=[]  KtParamMin=[]  KtParamMax=[]  POutMin=[]  POutMax=[]  IOutMin=[]  IOutMax=[]  DOutMin=[]  DOutMax=[]  NOutMin=[]  NOutMax=[]  KbOutMin=[]  KbOutMax=[]  KtOutMin=[]  KtOutMax=[]  IntegratorOutMin=[]  IntegratorOutMax=[]  FilterOutMin=[]  FilterOutMax=[]  SumOutMin=[]  SumOutMax=[]  SumI1OutMin=[]  SumI1OutMax=[]  SumI2OutMin=[]  SumI2OutMax=[]  SumI3OutMin=[]  SumI3OutMax=[]  SumDOutMin=[]  SumDOutMax=[]  SaturationOutMin=[]  SaturationOutMax=[]  IntegratorContinuousStateAttributes=''  IntegratorStateMustResolveToSignalObject=off  IntegratorRTWStateStorageClass=Auto  FilterContinuousStateAttributes=''  FilterStateMustResolveToSignalObject=off  FilterRTWStateStorageClass=Auto  DifferentiatorICPrevScaledInput=0  DifferentiatorOutMin=[]  DifferentiatorOutMax=[]  InitialConditionSetting=State (most efficient)
  cfblk6 : UnitDelay  SampleTime=-1
  cfblk7 : Delay  DelayLengthSource=Input port
      settings: InputPortMap=u0,p1
  cfblk8 : Delay  ShowEnablePort=on
      settings: InputPortMap=u0,e6
  cfblk9 : If  SampleTime=1
  cfblk2 : Outport
  cfblk12 : Outport  Port=2
  wires:
  cfblk6/1 -> cfblk2/1
  cfblk3/1 -> cfblk5/1
  cfblk10/1 -> cfblk13/1(cfblk1)
  cfblk7/1 -> cfblk8/1, cfblk12/1
  cfblk11/1 -> cfblk6/1
  cfblk8/1 -> cfblk4/1
  cfblk5/1 -> cfblk7/1, cfblk17/1
  cfblk1/1 -> cfblk14/1(cfblk1)
  cfblk14/1(cfblk2) -> cfblk8/2
  cfblk14/2(cfblk13) -> cfblk7/2
  cfblk14/3(cfblk14) -> cfblk3/1
  cfblk9/1 -> cfblk13/Action
  cfblk9/2 -> cfblk14/Action
  cfblk4/1 -> cfblk15/1
  cfblk15/1 -> cfblk13/2(cfblk10)
  cfblk13/1(cfblk2) -> cfblk16/1
  cfblk16/1 -> cfblk9/1
  cfblk17/1 -> cfblk14/2(cfblk12)

== system sampleModel2438/cfblk236 ==
  cfblk1 : Inport
  cfblk10 : Inport  Port=2
  Action Port : ActionPort  ActionType=then
  cfblk3 : simulink/Discrete/Transfer Fcn First Order  PoleZ=0.95  ICPrevOutput=0.0  DoSatur=off
      settings: SourceProductName=Simulink
  cfblk4 : Delay
  cfblk5 : simulink/Continuous/PID Controller  Controller=PID  TimeDomain=Discrete-time  SampleTime=-1  IntegratorMethod=Forward Euler  FilterMethod=Forward Euler  Form=Parallel  UseFilter=on  ControllerParametersSource=internal  P=1  I=1  D=0  N=100  InitialConditionSource=internal  InitialConditionForIntegrator=0  InitialConditionForFilter=0  ExternalReset=none  LimitOutput=off  UpperSaturationLimit=inf  LowerSaturationLimit=-inf  LinearizeAsGain=off  AntiWindupMode=none  Kb=1  TrackingMode=off  Kt=1  PParamMin=[]  PParamMax=[]  IParamMin=[]  IParamMax=[]  DParamMin=[]  DParamMax=[]  NParamMin=[]  NParamMax=[]  KbParamMin=[]  KbParamMax=[]  KtParamMin=[]  KtParamMax=[]  POutMin=[]  POutMax=[]  IOutMin=[]  IOutMax=[]  DOutMin=[]  DOutMax=[]  NOutMin=[]  NOutMax=[]  KbOutMin=[]  KbOutMax=[]  KtOutMin=[]  KtOutMax=[]  IntegratorOutMin=[]  IntegratorOutMax=[]  FilterOutMin=[]  FilterOutMax=[]  SumOutMin=[]  SumOutMax=[]  SumI1OutMin=[]  SumI1OutMax=[]  SumI2OutMin=[]  SumI2OutMax=[]  SumI3OutMin=[]  SumI3OutMax=[]  SumDOutMin=[]  SumDOutMax=[]  SaturationOutMin=[]  SaturationOutMax=[]  IntegratorContinuousStateAttributes=''  IntegratorStateMustResolveToSignalObject=off  IntegratorRTWStateStorageClass=Auto  FilterContinuousStateAttributes=''  FilterStateMustResolveToSignalObject=off  FilterRTWStateStorageClass=Auto  DifferentiatorICPrevScaledInput=0  DifferentiatorOutMin=[]  DifferentiatorOutMax=[]  InitialConditionSetting=State (most efficient)
  cfblk6 : DiscreteIntegrator  InitialConditionSetting=State (most efficient)  SampleTime=-1  ICPrevOutput=DiscIntNeverNeededParam  ICPrevScaledInput=DiscIntNeverNeededParam
  cfblk7 : simulink/Continuous/PID Controller  Controller=PID  TimeDomain=Discrete-time  SampleTime=-1  IntegratorMethod=Forward Euler  FilterMethod=Forward Euler  Form=Parallel  UseFilter=on  ControllerParametersSource=internal  P=1  I=1  D=0  N=100  InitialConditionSource=internal  InitialConditionForIntegrator=0  InitialConditionForFilter=0  ExternalReset=none  LimitOutput=off  UpperSaturationLimit=inf  LowerSaturationLimit=-inf  LinearizeAsGain=off  AntiWindupMode=none  Kb=1  TrackingMode=off  Kt=1  PParamMin=[]  PParamMax=[]  IParamMin=[]  IParamMax=[]  DParamMin=[]  DParamMax=[]  NParamMin=[]  NParamMax=[]  KbParamMin=[]  KbParamMax=[]  KtParamMin=[]  KtParamMax=[]  POutMin=[]  POutMax=[]  IOutMin=[]  IOutMax=[]  DOutMin=[]  DOutMax=[]  NOutMin=[]  NOutMax=[]  KbOutMin=[]  KbOutMax=[]  KtOutMin=[]  KtOutMax=[]  IntegratorOutMin=[]  IntegratorOutMax=[]  FilterOutMin=[]  FilterOutMax=[]  SumOutMin=[]  SumOutMax=[]  SumI1OutMin=[]  SumI1OutMax=[]  SumI2OutMin=[]  SumI2OutMax=[]  SumI3OutMin=[]  SumI3OutMax=[]  SumDOutMin=[]  SumDOutMax=[]  SaturationOutMin=[]  SaturationOutMax=[]  IntegratorContinuousStateAttributes=''  IntegratorStateMustResolveToSignalObject=off  IntegratorRTWStateStorageClass=Auto  FilterContinuousStateAttributes=''  FilterStateMustResolveToSignalObject=off  FilterRTWStateStorageClass=Auto  DifferentiatorICPrevScaledInput=0  DifferentiatorOutMin=[]  DifferentiatorOutMax=[]  InitialConditionSetting=State (most efficient)
  cfblk8 : Delay  ShowEnablePort=on
      settings: InputPortMap=u0,e6
  cfblk9 : DiscreteTransferFcn
  cfblk2 : Outport
  cfblk11 : Outport  Port=2
  cfblk12 : Outport  Port=3
  wires:
  cfblk9/1 -> cfblk12/1, cfblk8/2
  cfblk6/1 -> cfblk2/1
  cfblk7/1 -> cfblk5/1
  cfblk8/1 -> cfblk3/1
  cfblk1/1 -> cfblk11/1, cfblk4/1
  cfblk4/1 -> cfblk9/1
  cfblk10/1 -> cfblk7/1
  cfblk5/1 -> cfblk8/1
  cfblk3/1 -> cfblk6/1

== system sampleModel2438/cfblk237 ==
  cfblk1 : Inport
  cfblk9 : Inport  Port=2
  Action Port : ActionPort  ActionType=else
  cfblk11 : Delay
  cfblk3 : DiscreteIntegrator  InitialConditionSetting=State (most efficient)  SampleTime=-1  ICPrevOutput=DiscIntNeverNeededParam  ICPrevScaledInput=DiscIntNeverNeededParam
  cfblk4 : simulink/Discrete/Transfer Fcn Real Zero  ZeroZ=0.75  ICPrevInput=0.0  DoSatur=off
      settings: SourceProductName=Simulink  SourceProductBaseCode=SL
  cfblk5 : Delay  DelayLengthSource=Input port
      settings: InputPortMap=u0,p1
  cfblk6 : DiscreteZeroPole  Poles=[0 0.5]  Gain=1  SampleTime=-1
  cfblk7 : simulink/Continuous/PID Controller  Controller=PID  TimeDomain=Discrete-time  SampleTime=-1  IntegratorMethod=Forward Euler  FilterMethod=Forward Euler  Form=Parallel  UseFilter=on  ControllerParametersSource=internal  P=1  I=1  D=0  N=100  InitialConditionSource=internal  InitialConditionForIntegrator=0  InitialConditionForFilter=0  ExternalReset=none  LimitOutput=off  UpperSaturationLimit=inf  LowerSaturationLimit=-inf  LinearizeAsGain=off  AntiWindupMode=none  Kb=1  TrackingMode=off  Kt=1  PParamMin=[]  PParamMax=[]  IParamMin=[]  IParamMax=[]  DParamMin=[]  DParamMax=[]  NParamMin=[]  NParamMax=[]  KbParamMin=[]  KbParamMax=[]  KtParamMin=[]  KtParamMax=[]  POutMin=[]  POutMax=[]  IOutMin=[]  IOutMax=[]  DOutMin=[]  DOutMax=[]  NOutMin=[]  NOutMax=[]  KbOutMin=[]  KbOutMax=[]  KtOutMin=[]  KtOutMax=[]  IntegratorOutMin=[]  IntegratorOutMax=[]  FilterOutMin=[]  FilterOutMax=[]  SumOutMin=[]  SumOutMax=[]  SumI1OutMin=[]  SumI1OutMax=[]  SumI2OutMin=[]  SumI2OutMax=[]  SumI3OutMin=[]  SumI3OutMax=[]  SumDOutMin=[]  SumDOutMax=[]  SaturationOutMin=[]  SaturationOutMax=[]  IntegratorContinuousStateAttributes=''  IntegratorStateMustResolveToSignalObject=off  IntegratorRTWStateStorageClass=Auto  FilterContinuousStateAttributes=''  FilterStateMustResolveToSignalObject=off  FilterRTWStateStorageClass=Auto  DifferentiatorICPrevScaledInput=0  DifferentiatorOutMin=[]  DifferentiatorOutMax=[]  InitialConditionSetting=State (most efficient)
  cfblk8 : simulink/Continuous/PID Controller  Controller=PID  TimeDomain=Discrete-time  SampleTime=-1  IntegratorMethod=Forward Euler  FilterMethod=Forward Euler  Form=Parallel  UseFilter=on  ControllerParametersSource=internal  P=1  I=1  D=0  N=100  InitialConditionSource=internal  InitialConditionForIntegrator=0  InitialConditionForFilter=0  ExternalReset=none  LimitOutput=off  UpperSaturationLimit=inf  LowerSaturationLimit=-inf  LinearizeAsGain=off  AntiWindupMode=none  Kb=1  TrackingMode=off  Kt=1  PParamMin=[]  PParamMax=[]  IParamMin=[]  IParamMax=[]  DParamMin=[]  DParamMax=[]  NParamMin=[]  NParamMax=[]  KbParamMin=[]  KbParamMax=[]  KtParamMin=[]  KtParamMax=[]  POutMin=[]  POutMax=[]  IOutMin=[]  IOutMax=[]  DOutMin=[]  DOutMax=[]  NOutMin=[]  NOutMax=[]  KbOutMin=[]  KbOutMax=[]  KtOutMin=[]  KtOutMax=[]  IntegratorOutMin=[]  IntegratorOutMax=[]  FilterOutMin=[]  FilterOutMax=[]  SumOutMin=[]  SumOutMax=[]  SumI1OutMin=[]  SumI1OutMax=[]  SumI2OutMin=[]  SumI2OutMax=[]  SumI3OutMin=[]  SumI3OutMax=[]  SumDOutMin=[]  SumDOutMax=[]  SaturationOutMin=[]  SaturationOutMax=[]  IntegratorContinuousStateAttributes=''  IntegratorStateMustResolveToSignalObject=off  IntegratorRTWStateStorageClass=Auto  FilterContinuousStateAttributes=''  FilterStateMustResolveToSignalObject=off  FilterRTWStateStorageClass=Auto  DifferentiatorICPrevScaledInput=0  DifferentiatorOutMin=[]  DifferentiatorOutMax=[]  InitialConditionSetting=State (most efficient)
  cfblk2 : Outport
  cfblk10 : Outport  Port=2
  wires:
  cfblk1/1 -> cfblk8/1
  cfblk5/1 -> cfblk4/1
  cfblk8/1 -> cfblk6/1, cfblk5/2
  cfblk9/1 -> cfblk5/1
  cfblk3/1 -> cfblk7/1
  cfblk6/1 -> cfblk2/1
  cfblk4/1 -> cfblk10/1
  cfblk7/1 -> cfblk11/1
  cfblk11/1 -> cfblk3/1
